simulink model "wiener"  (R2019b)
settings: Solver=VariableStepAuto  StartTime=0.0  StopTime=stopTime  RelTol=1e-3
InitFcn:
  | Init;
StopFcn:
  | load('meansVect.mat');
  | meansOutVect = out.meansVect.signals.values;
undefined symbols (not defined in the file or in its folder): Ts_system, win
libraries: simulink x3
settings Model: Creator=cb54103  LastModifiedBy=Showi

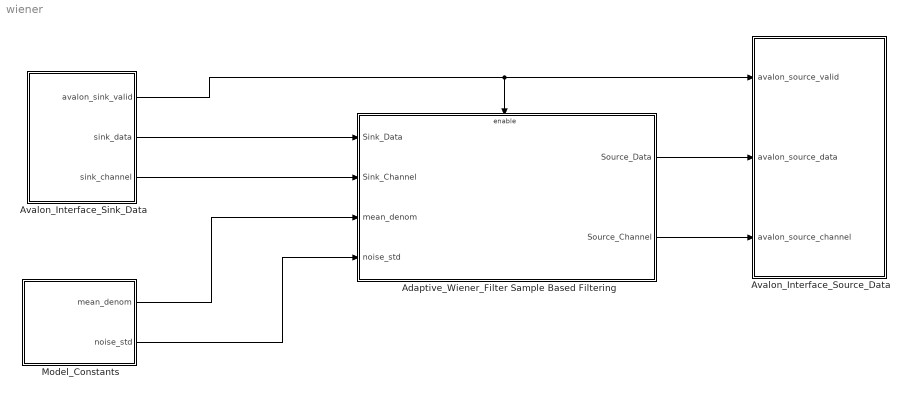
== system wiener ==
  Adaptive_Wiener_Filter Sample Based Filtering : Subsystem
  Avalon_Interface_Sink_Data : Subsystem
  Avalon_Interface_Source_Data : Subsystem
  Model_Constants : Subsystem
  wires:
  Adaptive_Wiener_Filter Sample Based Filtering/1(Source_Data) -> Avalon_Interface_Source_Data/2(avalon_source_data)
  Adaptive_Wiener_Filter Sample Based Filtering/2(Source_Channel) -> Avalon_Interface_Source_Data/3(avalon_source_channel)
  Avalon_Interface_Sink_Data/2(sink_data) -> Adaptive_Wiener_Filter Sample Based Filtering/1(Sink_Data)
  Avalon_Interface_Sink_Data/3(sink_channel) -> Adaptive_Wiener_Filter Sample Based Filtering/2(Sink_Channel)
  Avalon_Interface_Sink_Data/1(avalon_sink_valid) -> Adaptive_Wiener_Filter Sample Based Filtering/Enable, Avalon_Interface_Source_Data/1(avalon_source_valid)
  Model_Constants/1(mean_denom) -> Adaptive_Wiener_Filter Sample Based Filtering/3(mean_denom)
  Model_Constants/2(noise_std) -> Adaptive_Wiener_Filter Sample Based Filtering/4(noise_std)

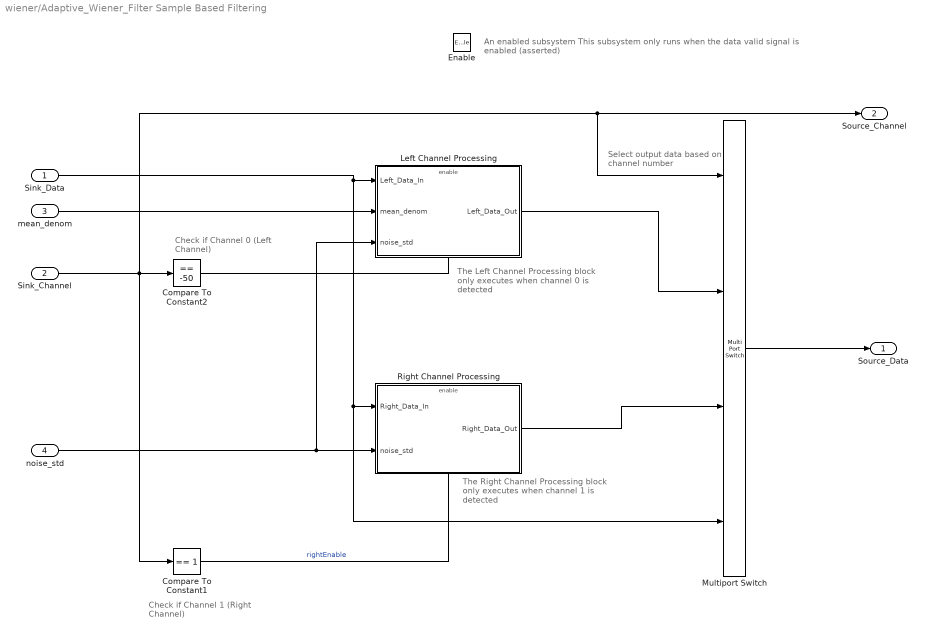
== system wiener/Adaptive_Wiener_Filter Sample Based Filtering ==
  note: The Left Channel Processing block
      | only executes when channel 0
      | is detected
  note: The Right Channel Processing block
      | only executes when channel 1
      | is detected
  note: Check if Channel 1
      | (Right Channel)
  note: Check if Channel 0
      | (Left Channel)
  note: Select output data
      | based on channel number
  note: An enabled subsystem
      | This subsystem only runs when the data valid signal is enabled (asserted)
  Sink_Data : Inport
  Sink_Channel : Inport  Port=2
  mean_denom : Inport  Port=3
  noise_std : Inport  Port=4
  Enable : EnablePort
  Compare To Constant1 : simulink/Logic and Bit Operations/Compare To Constant  relop===  const=1  OutDataTypeStr=boolean
  Compare To Constant2 : simulink/Logic and Bit Operations/Compare To Constant  relop===  const=-50  OutDataTypeStr=boolean
  Left Channel Processing : Subsystem  TreatAsAtomicUnit=on
  Multiport Switch : MultiPortSwitch  DataPortOrder=Zero-based contiguous  zeroidx=on
  Right Channel Processing : Subsystem  TreatAsAtomicUnit=on
  Source_Data : Outport  InitialOutput=0  VectorParamsAs1DForOutWhenUnconnected=off
  Source_Channel : Outport  Port=2  InitialOutput=0  VectorParamsAs1DForOutWhenUnconnected=off
  wires:
  Left Channel Processing/1("Left_Data_Out ") -> Multiport Switch/2
  Multiport Switch/1 -> Source_Data/1
  Compare To Constant2/1 -> Left Channel Processing/Enable
  Sink_Data/1 -> Multiport Switch/4, Right Channel Processing/1(Right_Data_In), Left Channel Processing/1(Left_Data_In)
  Right Channel Processing/1("Right_Data_Out ") -> Multiport Switch/3
  Sink_Channel/1 -> Source_Channel/1, Multiport Switch/1, Compare To Constant1/1, Compare To Constant2/1
  Compare To Constant1/1 -> Right Channel Processing/Enable  "rightEnable"
  mean_denom/1 -> Left Channel Processing/2(mean_denom)
  noise_std/1 -> Left Channel Processing/3(noise_std), Right Channel Processing/2(noise_std)

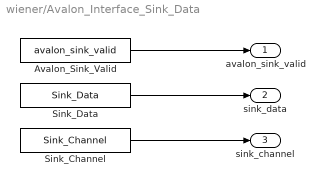
== system wiener/Avalon_Interface_Sink_Data ==
  Avalon_Sink_Valid : FromWorkspace  VariableName=avalon_sink_valid  SampleTime=Ts_system
  Sink_Channel : FromWorkspace  VariableName=Sink_Channel  SampleTime=Ts_system
  Sink_Data : FromWorkspace  VariableName=Sink_Data  SampleTime=Ts_system
  avalon_sink_valid : Outport  InitialOutput=0  VectorParamsAs1DForOutWhenUnconnected=off
  sink_data : Outport  Port=2  InitialOutput=0  VectorParamsAs1DForOutWhenUnconnected=off
  sink_channel : Outport  Port=3  InitialOutput=0  VectorParamsAs1DForOutWhenUnconnected=off
  wires:
  Sink_Channel/1 -> sink_channel/1
  Avalon_Sink_Valid/1 -> avalon_sink_valid/1
  Sink_Data/1 -> sink_data/1

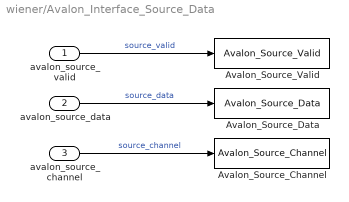
== system wiener/Avalon_Interface_Source_Data ==
  avalon_source_valid : Inport
  avalon_source_data : Inport  Port=2
  avalon_source_channel : Inport  Port=3
  Avalon_Source_Channel : ToWorkspace  VariableName=Avalon_Source_Channel  SaveFormat=Timeseries  SampleTime=-1
  Avalon_Source_Data : ToWorkspace  VariableName=Avalon_Source_Data  SaveFormat=Timeseries  SampleTime=-1
  Avalon_Source_Valid : ToWorkspace  VariableName=Avalon_Source_Valid  SaveFormat=Timeseries  SampleTime=-1
  wires:
  avalon_source_valid/1 -> Avalon_Source_Valid/1  "source_valid"
  avalon_source_data/1 -> Avalon_Source_Data/1  "source_data"
  avalon_source_channel/1 -> Avalon_Source_Channel/1  "source_channel"

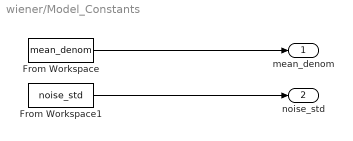
== system wiener/Model_Constants ==
  From Workspace : FromWorkspace  VariableName=mean_denom  SampleTime=Ts_system
  From Workspace1 : FromWorkspace  VariableName=noise_std  SampleTime=Ts_system
  mean_denom : Outport
  noise_std : Outport  Port=2
  wires:
  From Workspace/1 -> mean_denom/1
  From Workspace1/1 -> noise_std/1

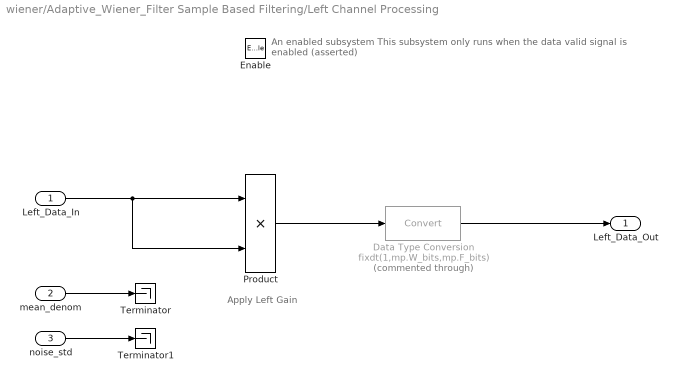
== system wiener/Adaptive_Wiener_Filter Sample Based Filtering/Left Channel Processing ==
  note: Apply Left Gain
  note: An enabled subsystem
      | This subsystem only runs when the data valid signal is enabled (asserted)
  Left_Data_In : Inport
  mean_denom : Inport  Port=2
  noise_std : Inport  Port=3
  Enable : EnablePort
  Data Type Conversion : DataTypeConversion  Commented=through  OutDataTypeStr=fixdt(1,mp.W_bits,mp.F_bits)
  Product : Product
  Terminator : Terminator
  Terminator1 : Terminator
  "Left_Data_Out " : Outport  InitialOutput=0  VectorParamsAs1DForOutWhenUnconnected=off
  wires:
  Product/1 -> Data Type Conversion/1
  Data Type Conversion/1 -> "Left_Data_Out "/1
  Left_Data_In/1 -> Product/2, Product/1
  mean_denom/1 -> Terminator/1
  noise_std/1 -> Terminator1/1

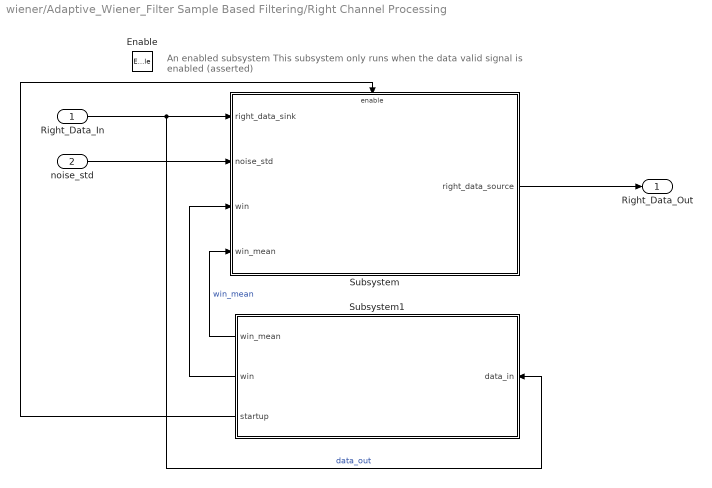
== system wiener/Adaptive_Wiener_Filter Sample Based Filtering/Right Channel Processing ==
  note: An enabled subsystem
      | This subsystem only runs when the data valid signal is enabled (asserted)
  Right_Data_In : Inport
  noise_std : Inport  Port=2
  Enable : EnablePort
  Subsystem : Subsystem
  Subsystem1 : Subsystem
  "Right_Data_Out " : Outport  InitialOutput=0  VectorParamsAs1DForOutWhenUnconnected=off
  wires:
  Right_Data_In/1 -> Subsystem1/1(data_in), Subsystem/1(right_data_sink)  "data_out"
  noise_std/1 -> Subsystem/2(noise_std)
  Subsystem/1(right_data_source) -> "Right_Data_Out "/1
  Subsystem1/1(win_mean) -> Subsystem/4(win_mean)  "win_mean"
  Subsystem1/2(win) -> Subsystem/3(win)
  Subsystem1/3(startup) -> Subsystem/Enable

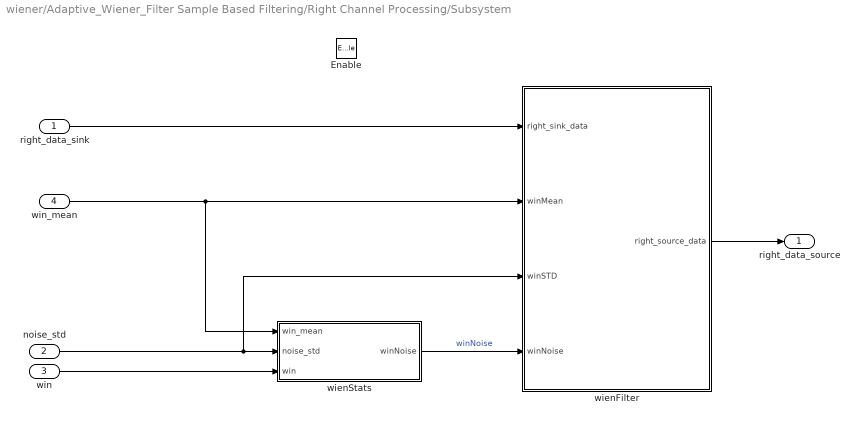
== system wiener/Adaptive_Wiener_Filter Sample Based Filtering/Right Channel Processing/Subsystem ==
  right_data_sink : Inport
  noise_std : Inport  Port=2
  win : Inport  Port=3
  win_mean : Inport  Port=4
  Enable : EnablePort
  wienFilter : Subsystem
  wienStats : Subsystem
  right_data_source : Outport
  wires:
  noise_std/1 -> wienFilter/3(winSTD), wienStats/2(noise_std)
  wienStats/1(winNoise) -> wienFilter/4(winNoise)  "winNoise"
  wienFilter/1(right_source_data) -> right_data_source/1
  win_mean/1 -> wienFilter/2(winMean), wienStats/1(win_mean)
  right_data_sink/1 -> wienFilter/1(right_sink_data)
  win/1 -> wienStats/3(win)

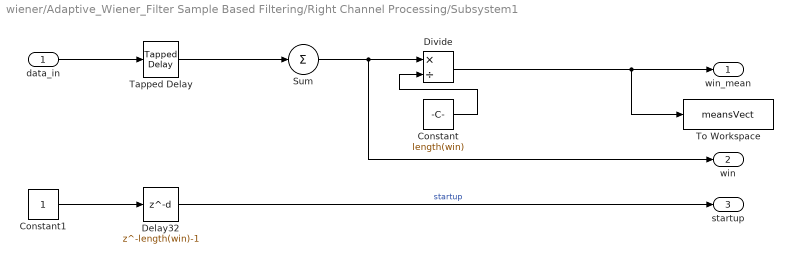
== system wiener/Adaptive_Wiener_Filter Sample Based Filtering/Right Channel Processing/Subsystem1 ==
  data_in : Inport
  Constant : Constant  Value=length(win)  SampleTime=-1
  Constant1 : Constant  SampleTime=-1
  Delay32 : Delay  DelayLength=length(win)-1
  Divide : Product  Inputs=*/
  Sum : Sum  Inputs=+
  Tapped Delay : simulink/Discrete/Tapped Delay  vinit=0.0  samptime=-1  NumDelays=length(win)-1  DelayOrder=Newest  includeCurrent=on
  To Workspace : ToWorkspace  VariableName=meansVect  SaveFormat=Structure With Time  SampleTime=-1
  win_mean : Outport
  win : Outport  Port=2
  startup : Outport  Port=3
  wires:
  data_in/1 -> Tapped Delay/1
  Tapped Delay/1 -> Sum/1
  Sum/1 -> win/1, Divide/1
  Constant/1 -> Divide/2
  Divide/1 -> To Workspace/1, win_mean/1
  Constant1/1 -> Delay32/1
  Delay32/1 -> startup/1  "startup"

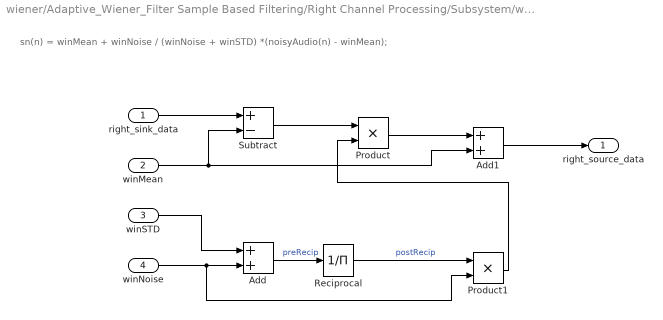
== system wiener/Adaptive_Wiener_Filter Sample Based Filtering/Right Channel Processing/Subsystem/wienFilter ==
  note: sn(n) = winMean + winNoise / (winNoise + winSTD) *(noisyAudio(n) - winMean);
  right_sink_data : Inport
  winMean : Inport  Port=2
  winSTD : Inport  Port=3
  winNoise : Inport  Port=4
  Add : Sum
  Add1 : Sum
  Product : Product
  Product1 : Product
  Reciprocal : Product  Inputs=/  SaturateOnIntegerOverflow=on  RndMeth=Zero
  Subtract : Sum  Inputs=+-
  right_source_data : Outport
  wires:
  winNoise/1 -> Product1/2, Add/2
  right_sink_data/1 -> Subtract/1
  winMean/1 -> Add1/2, Subtract/2
  Subtract/1 -> Product/1
  winSTD/1 -> Add/1
  Add/1 -> Reciprocal/1  "preRecip"
  Reciprocal/1 -> Product1/1  "postRecip"
  Product1/1 -> Product/2
  Product/1 -> Add1/1
  Add1/1 -> right_source_data/1

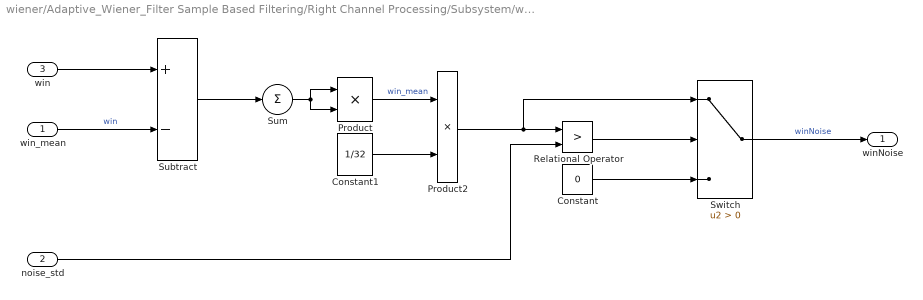
== system wiener/Adaptive_Wiener_Filter Sample Based Filtering/Right Channel Processing/Subsystem/wienStats ==
  win_mean : Inport
  noise_std : Inport  Port=2
  win : Inport  Port=3
  Constant : Constant  Value=0  SampleTime=-1
  Constant1 : Constant  Value=1/32  SampleTime=-1
  Product : Product
  Product2 : Product
  Relational Operator : RelationalOperator  Operator=>  OutDataTypeStr=boolean  RndMeth=Nearest
  Subtract : Sum  Inputs=+-
  Sum : Sum  Inputs=+
  Switch : Switch  Criteria=u2 > Threshold
  winNoise : Outport
  wires:
  Switch/1 -> winNoise/1  "winNoise"
  Constant1/1 -> Product2/2
  Subtract/1 -> Sum/1
  win/1 -> Subtract/1
  win_mean/1 -> Subtract/2  "win"
  Sum/1 -> Product/2, Product/1
  Product/1 -> Product2/1  "win_mean"
  noise_std/1 -> Relational Operator/2
  Product2/1 -> Switch/1, Relational Operator/1
  Relational Operator/1 -> Switch/2
  Constant/1 -> Switch/3
